simulink model "spoco12_100"  (R2013a)
settings: Solver=VariableStepDiscrete  SolverMode=SingleTasking  StartTime=0.0  StopTime=10.0  RelTol=1e-3
undefined symbols (not defined in the file or in its folder): casper_library_multipliers, cmult_4bit_em, pfb_coeff_gen_calc
libraries: xbsIndex_r4 x13471, casper_library_misc x184, xps_library x110, casper_library_delays x31
(part 3 of 135)

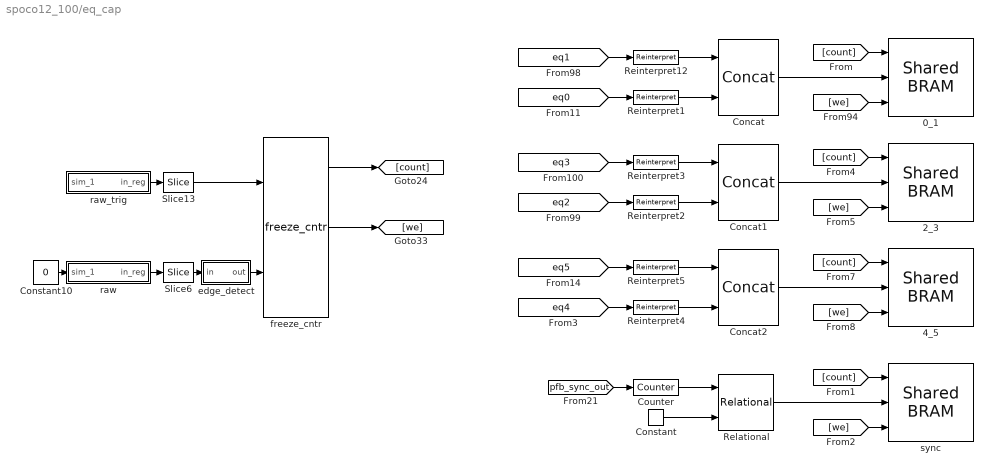
== system spoco12_100/eq_cap ==
  0_1 : xps_library/Shared BRAM  Tag=xps:bram  arith_type=Unsigned  addr_width=size+1  data_width=32  reg_prim_output=off  reg_core_output=off  optimization=Minimum_Area  data_bin_pt=0  init_vals=[1:2^10-1]  sample_rate=1
  2_3 : xps_library/Shared BRAM  Tag=xps:bram  arith_type=Unsigned  addr_width=size+1  data_width=32  reg_prim_output=off  reg_core_output=off  optimization=Minimum_Area  data_bin_pt=0  init_vals=[1:2^10-1]  sample_rate=1
  4_5 : xps_library/Shared BRAM  Tag=xps:bram  arith_type=Unsigned  addr_width=size+1  data_width=32  reg_prim_output=off  reg_core_output=off  optimization=Minimum_Area  data_bin_pt=0  init_vals=[1:2^10-1]  sample_rate=1
  Concat : xbsIndex_r4/Concat  num_inputs=2  dbl_ovrd=off  block_type=concat
  Concat1 : xbsIndex_r4/Concat  num_inputs=2  dbl_ovrd=off  block_type=concat
  Concat2 : xbsIndex_r4/Concat  num_inputs=2  dbl_ovrd=off  block_type=concat
  Constant : xbsIndex_r4/Constant  const=0  gui_display_data_type=Fixed-point  arith_type=Unsigned  n_bits=size  bin_pt=0  preci_type=Single  exp_width=8  frac_width=24  explicit_period=on  period=1  equ=P=C  opselect=C  inp2=PCIN>>17  opr=+  inp1=P  carry=CIN  dbl_ovrd=off  block_type=constant
  Constant10 : Constant  Value=0
  Counter : xbsIndex_r4/Counter  cnt_type=Free Running  cnt_to=Inf  operation=Up  start_count=0  cnt_by_val=1  arith_type=Unsigned  n_bits=size  bin_pt=0  load_pin=off  rst=on  en=off  explicit_period=on  period=1  use_behavioral_HDL=off  implementation=Fabric  dbl_ovrd=off  block_type=counter
  Reinterpret{1..5,12} (6 alike) : xbsIndex_r4/Reinterpret  force_arith_type=on  arith_type=Unsigned  force_bin_pt=on  bin_pt=0  block_type=reinterpret
  Relational : xbsIndex_r4/Relational  mode=a=b  op_type=Ufix  en=off  latency=0  dbl_ovrd=off  block_type=relational
  Slice13 : xbsIndex_r4/Slice  nbits=3  boolean_output=on  mode=Lower Bit Location + Width  bit1=0  base1=MSB of Input  bit0=0  base0=LSB of Input  dbl_ovrd=off  block_type=slice
  Slice6 : xbsIndex_r4/Slice  nbits=3  boolean_output=on  mode=Lower Bit Location + Width  bit1=0  base1=MSB of Input  bit0=0  base0=LSB of Input  dbl_ovrd=off  block_type=slice
  edge_detect : Subsystem  AncestorBlock=casper_library_misc/edge_detect  mask(edge_detect){edge=Both, polarity=Active High, x_in=[0 0.08 0.08 0.16 0.16 0.24 0.24 0.32 0.32 0.4], y_in=[-1 -1  1  1  1  1  1  1  1  1], x_out=[0.6 0.68 0.68 0.76 0.76 0.84 0.84 0.92 0.92 1], y_out=[-1 -1  1  1 -1 -1 -1 -1 -1 -1]}
      mask prompts: edge "Edge Type"; polarity "Output Polarity"; x_in "Input X Positions"; y_in "Input Y Positions"; x_out "Output X Positions"; y_out "Output Y Positions"
      mask help: Output is active for one-cycle after each edge of the specified type (i.e. rising, falling or both).
      mask init: same as spoco12_100/Sync/edge_detect1
      settings: AttributesFormatString=|
      | both edges
      | active high
      mask Help: Output is active for one-cycle after each edge of the specified type (i.e. rising, falling, or both).  Latency is zero.
      mask TypeOptions edge: Rising | Falling | Both
      mask TypeOptions polarity: Active High | Active Low
      mask Display:
      | plot(x_in_num,0.5+y_in_num*0.2);
      | plot(x_out_num,0.5+y_out_num*0.2);
  freeze_cntr : casper_library_misc/freeze_cntr  CounterBits=size+1
  raw : Subsystem  Tag=xps:sw_reg  AncestorBlock=xps_library/software register  mask(swreg){mode=one value, io_dir=From Processor, io_delay=0, sample_period=1, names=reg, bitwidths=32, arith_types=0, bin_pts=0, sim_port=on, show_format=off}
      mask prompts: io_dir "I/O direction"; io_delay "I/O delay"; sample_period "Sample period"; names "Name:"; bitwidths "Bitwidth:"; arith_types "Type (ufix=0, fix=1, bool=2):"; bin_pts "Binary pt:"; sim_port "Provide sim input/output?"; show_format "Print format string?"
      mask init:
      | swreg_init(gcb)
      settings: AttributesFormatString=1input
      mask TypeOptions mode: one value | fields of equal size | fields of arbitrary size
      mask Callback mode: swreg_cb(gcb);
      mask TypeOptions io_dir: To Processor | From Processor
      mask Callback io_dir:
      | mask_enables = get_param(gcb, 'MaskEnables');
      | mask_names = get_param(gcb, 'MaskNames');
      | if strcmp(get_param(gcb, 'io_dir'), 'To Processor'),
      |     mask_enables{ismember(mask_names, 'sample_period')} = 'off';
      | else
      |     mask_enables{ismember(mask_names, 'sample_period')} = 'on';
      | end
      | set_param(gcb, 'MaskEnables', mask_enables);
      mask Callback bitwidths:
      | swreg_maskcheck(gcb);
      | % blk = gcb;
      | % mode = get_param(blk, 'mode');
      | % current_widths = eval(get_param(blk, 'bitwidths'));
      | % if (strcmp(mode, 'one value') || strcmp(mode, 'fields of equal size')) && (length(current_widths) > 1),
      | %     error('Only one width may be specified for this mode.');
      | % elseif strcmp(mode, 'fields of arbitrary size')
      | %     current_names = textscan(strtrim(strrep(strrep(get_param(blk, 'names'), ']', ''), '[', '')), '%s');
      | %     current_names = current_names{1};
      | %     numios = length(current_names);
      | %     if length(current_widths) ~= numios,
      | %         error('%d field names specified, but %d widths?', numios, length(current_widths));
      | %     end
      | % end
      | % total_width = 0;
      | % for ctr = 1 : length(current_widths),
      | %     total_width = total_width + current_widths(ctr);
      | % end
      | % if total_width > 32,
      | %     error('Total width must be 32 or less, set to %d.', total_width);
      | % end
      mask Callback arith_types:
      | [numios, ~, ~, ~, current_types] = swreg_maskcheck(gcb);
      | % blk = gcb;
      | % mode = get_param(blk, 'mode');
      | % current_types = eval(get_param(blk, 'arith_types'));
      | % numios = length(current_types);
      | % if (strcmp(mode, 'one value') || strcmp(mode, 'fields of equal size')) && (length(current_types) > 1),
      | %     error('Only one type may be specified for this mode.');
      | % elseif strcmp(mode, 'fields of arbitrary size')
      | %     current_names = textscan(strtrim(strrep(strrep(get_param(blk, 'names'), ']', ''), '[', '')), '%s');
      | %     current_names = current_names{1};
      | %     numios = length(current_names);
      | %     if length(current_types) ~= numios,
      | %         error('%d field names specified, but %d types?', numios, length(current_types));
      | %     end
      | % end
      | problem = 0;
      | for ctr = 1 : numios,
      |     t = current_types(ctr);
      |     if (t < 0) || (t > 2),
      |         problem = t;
      |         ctr = numios + 1;
      |     end
      | end
      | if problem ~= 0,
      |     error('Type cannot be %i, must be 0, 1 or 2.', problem);
      | end
      mask Callback bin_pts:
      | swreg_maskcheck(gcb);
      | % blk = gcb;
      | % mode = get_param(blk, 'mode');
      | % current_bins = eval(get_param(blk, 'bin_pts'));
      | % if (strcmp(mode, 'one value') || strcmp(mode, 'fields of equal size')) && (length(current_bins) > 1),
      | %     error('Only one binary pt may be specified for this mode.');
      | % elseif strcmp(mode, 'fields of arbitrary size')
      | %     current_names = textscan(strtrim(strrep(strrep(get_param(blk, 'names'), ']', ''), '[', '')), '%s');
      | %     current_names = current_names{1};
      | %     numios = length(current_names);
      | %     if length(current_bins) ~= numios,
      | %         error('%d field names specified, but %d binary pts?', numios, length(current_bins));
      | %     end
      | % end
  raw_trig : Subsystem  Tag=xps:sw_reg  AncestorBlock=xps_library/software register  mask(swreg){mode=one value, io_dir=From Processor, io_delay=0, sample_period=1, names=reg, bitwidths=32, arith_types=0, bin_pts=0, sim_port=on, show_format=off}
      mask prompts: io_dir "I/O direction"; io_delay "I/O delay"; sample_period "Sample period"; names "Name:"; bitwidths "Bitwidth:"; arith_types "Type (ufix=0, fix=1, bool=2):"; bin_pts "Binary pt:"; sim_port "Provide sim input/output?"; show_format "Print format string?"
      mask init:
      | swreg_init(gcb)
      settings: AttributesFormatString=1input
      mask TypeOptions mode: one value | fields of equal size | fields of arbitrary size
      mask Callback mode: swreg_cb(gcb);
      mask TypeOptions io_dir: To Processor | From Processor
      mask Callback io_dir:
      | mask_enables = get_param(gcb, 'MaskEnables');
      | mask_names = get_param(gcb, 'MaskNames');
      | if strcmp(get_param(gcb, 'io_dir'), 'To Processor'),
      |     mask_enables{ismember(mask_names, 'sample_period')} = 'off';
      | else
      |     mask_enables{ismember(mask_names, 'sample_period')} = 'on';
      | end
      | set_param(gcb, 'MaskEnables', mask_enables);
      mask Callback bitwidths:
      | swreg_maskcheck(gcb);
      | % blk = gcb;
      | % mode = get_param(blk, 'mode');
      | % current_widths = eval(get_param(blk, 'bitwidths'));
      | % if (strcmp(mode, 'one value') || strcmp(mode, 'fields of equal size')) && (length(current_widths) > 1),
      | %     error('Only one width may be specified for this mode.');
      | % elseif strcmp(mode, 'fields of arbitrary size')
      | %     current_names = textscan(strtrim(strrep(strrep(get_param(blk, 'names'), ']', ''), '[', '')), '%s');
      | %     current_names = current_names{1};
      | %     numios = length(current_names);
      | %     if length(current_widths) ~= numios,
      | %         error('%d field names specified, but %d widths?', numios, length(current_widths));
      | %     end
      | % end
      | % total_width = 0;
      | % for ctr = 1 : length(current_widths),
      | %     total_width = total_width + current_widths(ctr);
      | % end
      | % if total_width > 32,
      | %     error('Total width must be 32 or less, set to %d.', total_width);
      | % end
      mask Callback arith_types:
      | [numios, ~, ~, ~, current_types] = swreg_maskcheck(gcb);
      | % blk = gcb;
      | % mode = get_param(blk, 'mode');
      | % current_types = eval(get_param(blk, 'arith_types'));
      | % numios = length(current_types);
      | % if (strcmp(mode, 'one value') || strcmp(mode, 'fields of equal size')) && (length(current_types) > 1),
      | %     error('Only one type may be specified for this mode.');
      | % elseif strcmp(mode, 'fields of arbitrary size')
      | %     current_names = textscan(strtrim(strrep(strrep(get_param(blk, 'names'), ']', ''), '[', '')), '%s');
      | %     current_names = current_names{1};
      | %     numios = length(current_names);
      | %     if length(current_types) ~= numios,
      | %         error('%d field names specified, but %d types?', numios, length(current_types));
      | %     end
      | % end
      | problem = 0;
      | for ctr = 1 : numios,
      |     t = current_types(ctr);
      |     if (t < 0) || (t > 2),
      |         problem = t;
      |         ctr = numios + 1;
      |     end
      | end
      | if problem ~= 0,
      |     error('Type cannot be %i, must be 0, 1 or 2.', problem);
      | end
      mask Callback bin_pts:
      | swreg_maskcheck(gcb);
      | % blk = gcb;
      | % mode = get_param(blk, 'mode');
      | % current_bins = eval(get_param(blk, 'bin_pts'));
      | % if (strcmp(mode, 'one value') || strcmp(mode, 'fields of equal size')) && (length(current_bins) > 1),
      | %     error('Only one binary pt may be specified for this mode.');
      | % elseif strcmp(mode, 'fields of arbitrary size')
      | %     current_names = textscan(strtrim(strrep(strrep(get_param(blk, 'names'), ']', ''), '[', '')), '%s');
      | %     current_names = current_names{1};
      | %     numios = length(current_names);
      | %     if length(current_bins) ~= numios,
      | %         error('%d field names specified, but %d binary pts?', numios, length(current_bins));
      | %     end
      | % end
  sync : xps_library/Shared BRAM  Tag=xps:bram  arith_type=Unsigned  addr_width=size+1  data_width=32  reg_prim_output=off  reg_core_output=off  optimization=Minimum_Area  data_bin_pt=0  init_vals=[1:2^10-1]  sample_rate=1
  wires:
  Constant/1 -> Relational/2
  Counter/1 -> Relational/1
  Relational/1 -> sync/2
  [pfb_sync_out] -> Counter/1
  [count] -> sync/1
  [we] -> sync/3
  raw/1(in_reg) -> Slice6/1
  freeze_cntr/1 -> [count]
  Slice6/1 -> edge_detect/1(in)
  freeze_cntr/2 -> [we]
  edge_detect/1(out) -> freeze_cntr/2
  raw_trig/1(in_reg) -> Slice13/1
  Slice13/1 -> freeze_cntr/1
  Constant10/1 -> raw/1(sim_1)
  Reinterpret1/1 -> Concat/2
  [eq1] -> Reinterpret12/1
  Reinterpret12/1 -> Concat/1
  Concat/1 -> 0_1/2
  [count] -> 0_1/1
  [we] -> 0_1/3
  [eq0] -> Reinterpret1/1
  Reinterpret2/1 -> Concat1/2
  Reinterpret3/1 -> Concat1/1
  Concat1/1 -> 2_3/2
  [count] -> 2_3/1
  [we] -> 2_3/3
  [eq2] -> Reinterpret2/1
  [eq3] -> Reinterpret3/1
  Reinterpret4/1 -> Concat2/2
  Reinterpret5/1 -> Concat2/1
  Concat2/1 -> 4_5/2
  [count] -> 4_5/1
  [we] -> 4_5/3
  [eq4] -> Reinterpret4/1
  [eq5] -> Reinterpret5/1

== system spoco12_100/eq_coeff ==
  sim_1 : Inport
  io_delay : xbsIndex_r4/Delay  rst=off  infoeditControl=Selection of Reset will increase slice count due to use of real FFs and instead of SRLs  en=off  latency=0  reg_retiming=on  dbl_ovrd=off  block_type=delay
  reint1 : xbsIndex_r4/Reinterpret  force_arith_type=on  arith_type=Unsigned  force_bin_pt=on  bin_pt=0  block_type=reinterpret
  slice_reg : xbsIndex_r4/Slice  nbits=32  boolean_output=off  mode=Lower Bit Location + Width  bit1=0  base1=MSB of Input  bit0=0  base0=LSB of Input  dbl_ovrd=off  block_type=slice
  spoco12_eq_coeff_user_data_out : xbsIndex_r4/Gateway In  gui_display_data_type=Fixed-point  arith_type=Unsigned  n_bits=32  bin_pt=0  preci_type=Single  exp_width=8  frac_width=24  rows=1  columns=1  quantization="Round  (unbiased: +/- Inf)"  overflow=Saturate  period=1  UseAsADC=off  ADCChannel='1'  interface=None  automatic_assignment=on  address_offset=hex2dec('00')  intf_description=''  timing_constraint=None  locs_specified=off  LOCs={}  io_standard={}  inherit_from_input=off  hdl_port=on  dbl_ovrd=off  block_type=gatewayin
  in_reg : Outport
  wires:
  spoco12_eq_coeff_user_data_out/1 -> io_delay/1
  sim_1/1 -> spoco12_eq_coeff_user_data_out/1
  io_delay/1 -> slice_reg/1
  slice_reg/1 -> reint1/1
  reint1/1 -> in_reg/1

== system spoco12_100/fft ==
  sync : Inport
  shift : Inport  Port=2
  pol0_in : Inport  Port=3
  pol1_in : Inport  Port=4
  pol2_in : Inport  Port=5
  pol3_in : Inport  Port=6
  pol4_in : Inport  Port=7
  pol5_in : Inport  Port=8
  pol6_in : Inport  Port=9
  pol7_in : Inport  Port=10
  pol8_in : Inport  Port=11
  pol9_in : Inport  Port=12
  pol10_in : Inport  Port=13
  pol11_in : Inport  Port=14
  fft_biplex_real_2x : Subsystem  Tag=casper:fft_biplex_real_2x  AncestorBlock=casper_library_ffts/fft_biplex_real_2x  mask(fft_biplex_real_2x){n_inputs=3, FFTSize=size, input_bit_width=18, bin_pt=17, coeff_bit_width=18, async=off, add_latency=add_z, mult_latency=mult_z, bram_latency=bram_z, conv_latency=cast_z, quantization=Round  (unbiased: +/- Inf), overflow=Saturate, delays_bit_limit=8, coeffs_bit_limit=8, coeff_sharing=on, coeff_decimation=on, max_fanout=4, mult_spec=2, bitgrowth=off, max_bits=19, hardcode_shifts=off, shift_schedule=[1                                      1], dsp48_adders=off}
      mask prompts: n_inputs "Number simultaneous inputs (4*?)"; FFTSize "Size of FFT: (2^? pts)"; input_bit_width "Input bit width"; bin_pt "Input binary point"; coeff_bit_width "Coefficient Bit Width"; async "Asynchronous operation"; add_latency "Add Latency"; mult_latency "Mult Latency"; bram_latency "BRAM Latency"; conv_latency "Convert latency"; quantization "Quantization Behavior"; overflow "Overflow Behavior"; delays_bit_limit "Number bits above which to implement stage's delays in BRAM (2^? bits)"; coeffs_bit_limit "Number bits above which to store stage's coefficients in BRAM (2^? bits)"; coeff_sharing "BRAM sharing in coeff storage"; coeff_decimation "Store a fraction of coeff factors where useful"; max_fanout "Maximum fanout"; mult_spec "Multiplier impl. (0=core, 1=embedded, 2=behavioural) (left=1st stage, or just one value)"; bitgrowth "Bit growth instead of shifting"; max_bits "Max bits to growth to"; hardcode_shifts "Hardcode shift schedule"; shift_schedule "Shift schedule"; dsp48_adders "DSP48 adders in butterfly"
      mask help: A real-sampled biplex FFT, with output demuxed by 2.
      mask init:
      | fft_biplex_real_2x_init(gcb, ...
      |     'n_inputs', n_inputs, ...
      |     'FFTSize', FFTSize, ...
      |     'input_bit_width', input_bit_width, ... 
      |     'bin_pt', bin_pt, ...
      |     'coeff_bit_width', coeff_bit_width, ...
      |     'async', async, ...
      |     'add_latency', add_latency, ...
      |     'mult_latency', mult_latency, ...
      |     'bram_latency', bram_latency, ...
      |     'conv_latency', conv_latency, ...
      |     'quantization', quantization, ...
      |     'overflow', overflow, ...
      |     'delays_bit_limit', delays_bit_limit, ...
      |     'coeffs_bit_limit', coeffs_bit_limit, ...
      |     'coeff_sharing', coeff_sharing, ...
      |     'coeff_decimation', coeff_decimation, ...
      |     'max_fanout', max_fanout, ...
      |     'mult_spec', mult_spec, ...
      |     'bitgrowth', bitgrowth, ...
      |     'max_bits', max_bits, ...
      |     'hardcode_shifts', hardcode_shifts, ...
      |     'shift_schedule', shift_schedule, ...
      |     'dsp48_adders', dsp48_adders);
      settings: AttributesFormatString=|
      | 10 stages
      | [18,18]
      | Round  (unbiased: +/- Inf)
      | Saturate
      mask Help: eval('xlWeb(''http://casper.berkeley.edu/wiki/Fft_biplex_real_2x'')')
      mask TypeOptions quantization: Truncate | Round  (unbiased: +/- Inf) | Round  (unbiased: Even Values)
      mask TypeOptions overflow: Wrap | Saturate | Error
      mask Callback hardcode_shifts:
      | hardcode_shifts = get_param(gcb, 'hardcode_shifts');
      | set_param_state(gcb, 'shift_schedule', hardcode_shifts);
      mask Callback dsp48_adders: fft_callback_dsp48_adders(gcb);
  sync_out : Outport
  pol02_out : Outport  Port=2
  pol13_out : Outport  Port=3
  pol46_out : Outport  Port=4
  pol57_out : Outport  Port=5
  pol810_out : Outport  Port=6
  pol911_out : Outport  Port=7
  of : Outport  Port=8
  wires:
  fft_biplex_real_2x/8(of) -> of/1
  shift/1 -> fft_biplex_real_2x/2(shift)
  sync/1 -> fft_biplex_real_2x/1(sync)
  fft_biplex_real_2x/1(sync_out) -> [sync_out], sync_out/1
  fft_biplex_real_2x/2(pol02_out) -> [pol02_out], pol02_out/1
  fft_biplex_real_2x/3(pol13_out) -> [pol13_out], pol13_out/1
  fft_biplex_real_2x/4(pol46_out) -> [pol46_out], pol46_out/1
  fft_biplex_real_2x/5(pol57_out) -> [pol57_out], pol57_out/1
  fft_biplex_real_2x/6(pol810_out) -> [pol810_out], pol810_out/1
  fft_biplex_real_2x/7(pol911_out) -> [pol911_out], pol911_out/1
  pol0_in/1 -> fft_biplex_real_2x/3(pol0_in)
  pol9_in/1 -> fft_biplex_real_2x/12(pol9_in)
  pol7_in/1 -> fft_biplex_real_2x/10(pol7_in)
  pol8_in/1 -> fft_biplex_real_2x/11(pol8_in)
  pol11_in/1 -> fft_biplex_real_2x/14(pol11_in)
  pol3_in/1 -> fft_biplex_real_2x/6(pol3_in)
  pol6_in/1 -> fft_biplex_real_2x/9(pol6_in)
  pol10_in/1 -> fft_biplex_real_2x/13(pol10_in)
  pol5_in/1 -> fft_biplex_real_2x/8(pol5_in)
  pol1_in/1 -> fft_biplex_real_2x/4(pol1_in)
  pol2_in/1 -> fft_biplex_real_2x/5(pol2_in)
  pol4_in/1 -> fft_biplex_real_2x/7(pol4_in)

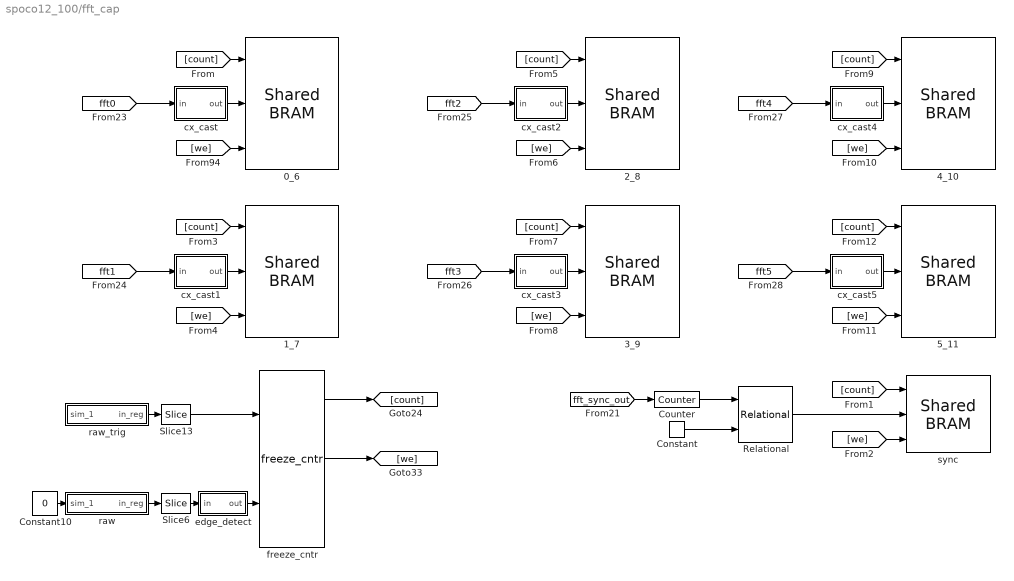
== system spoco12_100/fft_cap ==
  0_6 : xps_library/Shared BRAM  Tag=xps:bram  arith_type=Unsigned  addr_width=size+1  data_width=32  reg_prim_output=off  reg_core_output=off  optimization=Minimum_Area  data_bin_pt=0  init_vals=[1:2^10-1]  sample_rate=1
  1_7 : xps_library/Shared BRAM  Tag=xps:bram  arith_type=Unsigned  addr_width=size+1  data_width=32  reg_prim_output=off  reg_core_output=off  optimization=Minimum_Area  data_bin_pt=0  init_vals=[1:2^10-1]  sample_rate=1
  2_8 : xps_library/Shared BRAM  Tag=xps:bram  arith_type=Unsigned  addr_width=size+1  data_width=32  reg_prim_output=off  reg_core_output=off  optimization=Minimum_Area  data_bin_pt=0  init_vals=[1:2^10-1]  sample_rate=1
  3_9 : xps_library/Shared BRAM  Tag=xps:bram  arith_type=Unsigned  addr_width=size+1  data_width=32  reg_prim_output=off  reg_core_output=off  optimization=Minimum_Area  data_bin_pt=0  init_vals=[1:2^10-1]  sample_rate=1
  4_10 : xps_library/Shared BRAM  Tag=xps:bram  arith_type=Unsigned  addr_width=size+1  data_width=32  reg_prim_output=off  reg_core_output=off  optimization=Minimum_Area  data_bin_pt=0  init_vals=[1:2^10-1]  sample_rate=1
  5_11 : xps_library/Shared BRAM  Tag=xps:bram  arith_type=Unsigned  addr_width=size+1  data_width=32  reg_prim_output=off  reg_core_output=off  optimization=Minimum_Area  data_bin_pt=0  init_vals=[1:2^10-1]  sample_rate=1
  Constant : xbsIndex_r4/Constant  const=0  gui_display_data_type=Fixed-point  arith_type=Unsigned  n_bits=size  bin_pt=0  preci_type=Single  exp_width=8  frac_width=24  explicit_period=on  period=1  equ=P=C  opselect=C  inp2=PCIN>>17  opr=+  inp1=P  carry=CIN  dbl_ovrd=off  block_type=constant
  Constant10 : Constant  Value=0
  Counter : xbsIndex_r4/Counter  cnt_type=Free Running  cnt_to=Inf  operation=Up  start_count=0  cnt_by_val=1  arith_type=Unsigned  n_bits=size  bin_pt=0  load_pin=off  rst=on  en=off  explicit_period=on  period=1  use_behavioral_HDL=off  implementation=Fabric  dbl_ovrd=off  block_type=counter
  Relational : xbsIndex_r4/Relational  mode=a=b  op_type=Ufix  en=off  latency=0  dbl_ovrd=off  block_type=relational
  Slice13 : xbsIndex_r4/Slice  nbits=3  boolean_output=on  mode=Lower Bit Location + Width  bit1=0  base1=MSB of Input  bit0=0  base0=LSB of Input  dbl_ovrd=off  block_type=slice
  Slice6 : xbsIndex_r4/Slice  nbits=3  boolean_output=on  mode=Lower Bit Location + Width  bit1=0  base1=MSB of Input  bit0=0  base0=LSB of Input  dbl_ovrd=off  block_type=slice
  cx_cast : Subsystem  mask{in_bits=18, in_bp=17, out_bits=16, out_bp=15}
      mask prompts: in_bits "Input bits"; in_bp "Input binary point"; out_bits "Output bits"; out_bp "Output binary point"
  cx_cast1 : Subsystem  mask{in_bits=18, in_bp=17, out_bits=16, out_bp=15}
      mask prompts: in_bits "Input bits"; in_bp "Input binary point"; out_bits "Output bits"; out_bp "Output binary point"
  cx_cast2 : Subsystem  mask{in_bits=18, in_bp=17, out_bits=16, out_bp=15}
      mask prompts: in_bits "Input bits"; in_bp "Input binary point"; out_bits "Output bits"; out_bp "Output binary point"
  cx_cast3 : Subsystem  mask{in_bits=18, in_bp=17, out_bits=16, out_bp=15}
      mask prompts: in_bits "Input bits"; in_bp "Input binary point"; out_bits "Output bits"; out_bp "Output binary point"
  cx_cast4 : Subsystem  mask{in_bits=18, in_bp=17, out_bits=16, out_bp=15}
      mask prompts: in_bits "Input bits"; in_bp "Input binary point"; out_bits "Output bits"; out_bp "Output binary point"
  cx_cast5 : Subsystem  mask{in_bits=18, in_bp=17, out_bits=16, out_bp=15}
      mask prompts: in_bits "Input bits"; in_bp "Input binary point"; out_bits "Output bits"; out_bp "Output binary point"
  edge_detect : Subsystem  AncestorBlock=casper_library_misc/edge_detect  mask(edge_detect){edge=Both, polarity=Active High, x_in=[0 0.08 0.08 0.16 0.16 0.24 0.24 0.32 0.32 0.4], y_in=[-1 -1  1  1  1  1  1  1  1  1], x_out=[0.6 0.68 0.68 0.76 0.76 0.84 0.84 0.92 0.92 1], y_out=[-1 -1  1  1 -1 -1 -1 -1 -1 -1]}
      mask prompts: edge "Edge Type"; polarity "Output Polarity"; x_in "Input X Positions"; y_in "Input Y Positions"; x_out "Output X Positions"; y_out "Output Y Positions"
      mask help: Output is active for one-cycle after each edge of the specified type (i.e. rising, falling or both).
      mask init: same as spoco12_100/Sync/edge_detect1
      settings: AttributesFormatString=|
      | both edges
      | active high
      mask Help: Output is active for one-cycle after each edge of the specified type (i.e. rising, falling, or both).  Latency is zero.
      mask TypeOptions edge: Rising | Falling | Both
      mask TypeOptions polarity: Active High | Active Low
      mask Display:
      | plot(x_in_num,0.5+y_in_num*0.2);
      | plot(x_out_num,0.5+y_out_num*0.2);
  freeze_cntr : casper_library_misc/freeze_cntr  CounterBits=size+1
  raw : Subsystem  Tag=xps:sw_reg  AncestorBlock=xps_library/software register  mask(swreg){mode=one value, io_dir=From Processor, io_delay=0, sample_period=1, names=reg, bitwidths=32, arith_types=0, bin_pts=0, sim_port=on, show_format=off}
      mask prompts: io_dir "I/O direction"; io_delay "I/O delay"; sample_period "Sample period"; names "Name:"; bitwidths "Bitwidth:"; arith_types "Type (ufix=0, fix=1, bool=2):"; bin_pts "Binary pt:"; sim_port "Provide sim input/output?"; show_format "Print format string?"
      mask init:
      | swreg_init(gcb)
      settings: AttributesFormatString=1input
      mask TypeOptions mode: one value | fields of equal size | fields of arbitrary size
      mask Callback mode: swreg_cb(gcb);
      mask TypeOptions io_dir: To Processor | From Processor
      mask Callback io_dir:
      | mask_enables = get_param(gcb, 'MaskEnables');
      | mask_names = get_param(gcb, 'MaskNames');
      | if strcmp(get_param(gcb, 'io_dir'), 'To Processor'),
      |     mask_enables{ismember(mask_names, 'sample_period')} = 'off';
      | else
      |     mask_enables{ismember(mask_names, 'sample_period')} = 'on';
      | end
      | set_param(gcb, 'MaskEnables', mask_enables);
      mask Callback bitwidths:
      | swreg_maskcheck(gcb);
      | % blk = gcb;
      | % mode = get_param(blk, 'mode');
      | % current_widths = eval(get_param(blk, 'bitwidths'));
      | % if (strcmp(mode, 'one value') || strcmp(mode, 'fields of equal size')) && (length(current_widths) > 1),
      | %     error('Only one width may be specified for this mode.');
      | % elseif strcmp(mode, 'fields of arbitrary size')
      | %     current_names = textscan(strtrim(strrep(strrep(get_param(blk, 'names'), ']', ''), '[', '')), '%s');
      | %     current_names = current_names{1};
      | %     numios = length(current_names);
      | %     if length(current_widths) ~= numios,
      | %         error('%d field names specified, but %d widths?', numios, length(current_widths));
      | %     end
      | % end
      | % total_width = 0;
      | % for ctr = 1 : length(current_widths),
      | %     total_width = total_width + current_widths(ctr);
      | % end
      | % if total_width > 32,
      | %     error('Total width must be 32 or less, set to %d.', total_width);
      | % end
      mask Callback arith_types:
      | [numios, ~, ~, ~, current_types] = swreg_maskcheck(gcb);
      | % blk = gcb;
      | % mode = get_param(blk, 'mode');
      | % current_types = eval(get_param(blk, 'arith_types'));
      | % numios = length(current_types);
      | % if (strcmp(mode, 'one value') || strcmp(mode, 'fields of equal size')) && (length(current_types) > 1),
      | %     error('Only one type may be specified for this mode.');
      | % elseif strcmp(mode, 'fields of arbitrary size')
      | %     current_names = textscan(strtrim(strrep(strrep(get_param(blk, 'names'), ']', ''), '[', '')), '%s');
      | %     current_names = current_names{1};
      | %     numios = length(current_names);
      | %     if length(current_types) ~= numios,
      | %         error('%d field names specified, but %d types?', numios, length(current_types));
      | %     end
      | % end
      | problem = 0;
      | for ctr = 1 : numios,
      |     t = current_types(ctr);
      |     if (t < 0) || (t > 2),
      |         problem = t;
      |         ctr = numios + 1;
      |     end
      | end
      | if problem ~= 0,
      |     error('Type cannot be %i, must be 0, 1 or 2.', problem);
      | end
      mask Callback bin_pts:
      | swreg_maskcheck(gcb);
      | % blk = gcb;
      | % mode = get_param(blk, 'mode');
      | % current_bins = eval(get_param(blk, 'bin_pts'));
      | % if (strcmp(mode, 'one value') || strcmp(mode, 'fields of equal size')) && (length(current_bins) > 1),
      | %     error('Only one binary pt may be specified for this mode.');
      | % elseif strcmp(mode, 'fields of arbitrary size')
      | %     current_names = textscan(strtrim(strrep(strrep(get_param(blk, 'names'), ']', ''), '[', '')), '%s');
      | %     current_names = current_names{1};
      | %     numios = length(current_names);
      | %     if length(current_bins) ~= numios,
      | %         error('%d field names specified, but %d binary pts?', numios, length(current_bins));
      | %     end
      | % end
  raw_trig : Subsystem  Tag=xps:sw_reg  AncestorBlock=xps_library/software register  mask(swreg){mode=one value, io_dir=From Processor, io_delay=0, sample_period=1, names=reg, bitwidths=32, arith_types=0, bin_pts=0, sim_port=on, show_format=off}
      mask prompts: io_dir "I/O direction"; io_delay "I/O delay"; sample_period "Sample period"; names "Name:"; bitwidths "Bitwidth:"; arith_types "Type (ufix=0, fix=1, bool=2):"; bin_pts "Binary pt:"; sim_port "Provide sim input/output?"; show_format "Print format string?"
      mask init:
      | swreg_init(gcb)
      settings: AttributesFormatString=1input
      mask TypeOptions mode: one value | fields of equal size | fields of arbitrary size
      mask Callback mode: swreg_cb(gcb);
      mask TypeOptions io_dir: To Processor | From Processor
      mask Callback io_dir:
      | mask_enables = get_param(gcb, 'MaskEnables');
      | mask_names = get_param(gcb, 'MaskNames');
      | if strcmp(get_param(gcb, 'io_dir'), 'To Processor'),
      |     mask_enables{ismember(mask_names, 'sample_period')} = 'off';
      | else
      |     mask_enables{ismember(mask_names, 'sample_period')} = 'on';
      | end
      | set_param(gcb, 'MaskEnables', mask_enables);
      mask Callback bitwidths:
      | swreg_maskcheck(gcb);
      | % blk = gcb;
      | % mode = get_param(blk, 'mode');
      | % current_widths = eval(get_param(blk, 'bitwidths'));
      | % if (strcmp(mode, 'one value') || strcmp(mode, 'fields of equal size')) && (length(current_widths) > 1),
      | %     error('Only one width may be specified for this mode.');
      | % elseif strcmp(mode, 'fields of arbitrary size')
      | %     current_names = textscan(strtrim(strrep(strrep(get_param(blk, 'names'), ']', ''), '[', '')), '%s');
      | %     current_names = current_names{1};
      | %     numios = length(current_names);
      | %     if length(current_widths) ~= numios,
      | %         error('%d field names specified, but %d widths?', numios, length(current_widths));
      | %     end
      | % end
      | % total_width = 0;
      | % for ctr = 1 : length(current_widths),
      | %     total_width = total_width + current_widths(ctr);
      | % end
      | % if total_width > 32,
      | %     error('Total width must be 32 or less, set to %d.', total_width);
      | % end
      mask Callback arith_types:
      | [numios, ~, ~, ~, current_types] = swreg_maskcheck(gcb);
      | % blk = gcb;
      | % mode = get_param(blk, 'mode');
      | % current_types = eval(get_param(blk, 'arith_types'));
      | % numios = length(current_types);
      | % if (strcmp(mode, 'one value') || strcmp(mode, 'fields of equal size')) && (length(current_types) > 1),
      | %     error('Only one type may be specified for this mode.');
      | % elseif strcmp(mode, 'fields of arbitrary size')
      | %     current_names = textscan(strtrim(strrep(strrep(get_param(blk, 'names'), ']', ''), '[', '')), '%s');
      | %     current_names = current_names{1};
      | %     numios = length(current_names);
      | %     if length(current_types) ~= numios,
      | %         error('%d field names specified, but %d types?', numios, length(current_types));
      | %     end
      | % end
      | problem = 0;
      | for ctr = 1 : numios,
      |     t = current_types(ctr);
      |     if (t < 0) || (t > 2),
      |         problem = t;
      |         ctr = numios + 1;
      |     end
      | end
      | if problem ~= 0,
      |     error('Type cannot be %i, must be 0, 1 or 2.', problem);
      | end
      mask Callback bin_pts:
      | swreg_maskcheck(gcb);
      | % blk = gcb;
      | % mode = get_param(blk, 'mode');
      | % current_bins = eval(get_param(blk, 'bin_pts'));
      | % if (strcmp(mode, 'one value') || strcmp(mode, 'fields of equal size')) && (length(current_bins) > 1),
      | %     error('Only one binary pt may be specified for this mode.');
      | % elseif strcmp(mode, 'fields of arbitrary size')
      | %     current_names = textscan(strtrim(strrep(strrep(get_param(blk, 'names'), ']', ''), '[', '')), '%s');
      | %     current_names = current_names{1};
      | %     numios = length(current_names);
      | %     if length(current_bins) ~= numios,
      | %         error('%d field names specified, but %d binary pts?', numios, length(current_bins));
      | %     end
      | % end
  sync : xps_library/Shared BRAM  Tag=xps:bram  arith_type=Unsigned  addr_width=size+1  data_width=32  reg_prim_output=off  reg_core_output=off  optimization=Minimum_Area  data_bin_pt=0  init_vals=[1:2^10-1]  sample_rate=1
  wires:
  Constant/1 -> Relational/2
  Counter/1 -> Relational/1
  Relational/1 -> sync/2
  [fft_sync_out] -> Counter/1
  [count] -> sync/1
  [we] -> sync/3
  raw/1(in_reg) -> Slice6/1
  freeze_cntr/1 -> [count]
  Slice6/1 -> edge_detect/1(in)
  freeze_cntr/2 -> [we]
  edge_detect/1(out) -> freeze_cntr/2
  raw_trig/1(in_reg) -> Slice13/1
  Slice13/1 -> freeze_cntr/1
  Constant10/1 -> raw/1(sim_1)
  [count] -> 0_6/1
  [we] -> 0_6/3
  [fft0] -> cx_cast/1(in)
  cx_cast/1(out) -> 0_6/2
  [count] -> 1_7/1
  [we] -> 1_7/3
  [fft1] -> cx_cast1/1(in)
  cx_cast1/1(out) -> 1_7/2
  [count] -> 2_8/1
  [we] -> 2_8/3
  [fft2] -> cx_cast2/1(in)
  cx_cast2/1(out) -> 2_8/2
  [count] -> 3_9/1
  [we] -> 3_9/3
  [fft3] -> cx_cast3/1(in)
  cx_cast3/1(out) -> 3_9/2
  [count] -> 4_10/1
  [we] -> 4_10/3
  [fft4] -> cx_cast4/1(in)
  cx_cast4/1(out) -> 4_10/2
  [count] -> 5_11/1
  [we] -> 5_11/3
  [fft5] -> cx_cast5/1(in)
  cx_cast5/1(out) -> 5_11/2

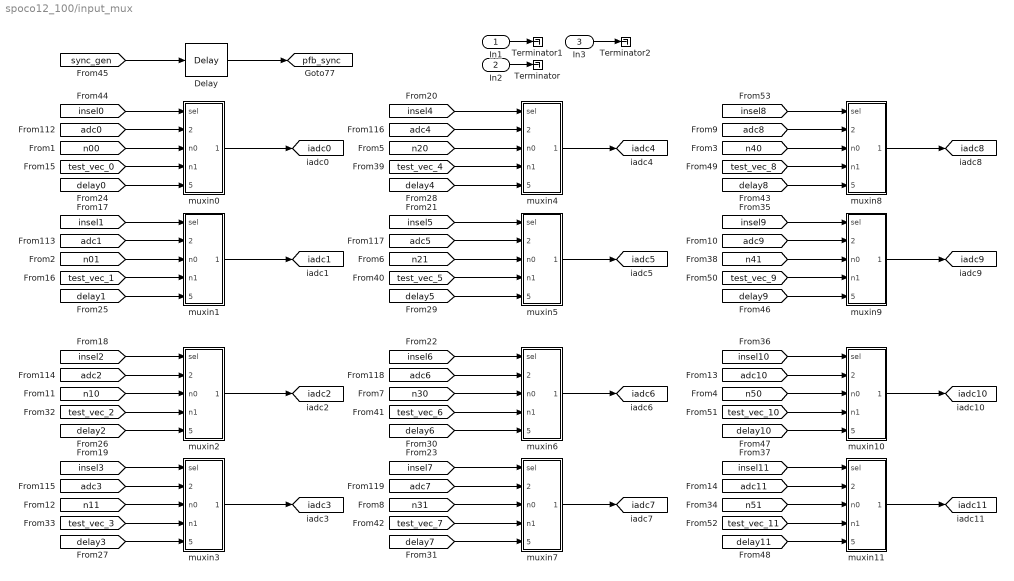
== system spoco12_100/input_mux ==
  In1 : Inport
  In2 : Inport  Port=2
  In3 : Inport  Port=3
  Delay : xbsIndex_r4/Delay  rst=off  infoeditControl=Selection of Reset will increase slice count due to use of real FFs and instead of SRLs  en=off  latency=2  reg_retiming=off  dbl_ovrd=off  block_type=delay
  Terminator : Terminator
  Terminator1 : Terminator
  Terminator2 : Terminator
  muxin0 : Subsystem
  muxin1 : Subsystem
  muxin10 : Subsystem
  muxin11 : Subsystem
  muxin2 : Subsystem
  muxin3 : Subsystem
  muxin4 : Subsystem
  muxin5 : Subsystem
  muxin6 : Subsystem
  muxin7 : Subsystem
  muxin8 : Subsystem
  muxin9 : Subsystem
  tag scope: iadc0=global, iadc10=global, iadc11=global, iadc1=global, iadc2=global, iadc3=global, iadc4=global, iadc5=global, iadc6=global, iadc7=global, iadc8=global, iadc9=global, pfb_sync=global
  wires:
  [insel0] -> muxin0/1(sel)
  [adc0] -> muxin0/2(adc)
  [n00] -> muxin0/3(n0)
  [delay0] -> muxin0/5(delay)
  [insel1] -> muxin1/1(sel)
  [adc1] -> muxin1/2(adc)
  [delay1] -> muxin1/5(delay)
  [insel2] -> muxin2/1(sel)
  [adc2] -> muxin2/2(adc)
  [n10] -> muxin2/3(n0)
  [delay2] -> muxin2/5(delay)
  [insel3] -> muxin3/1(sel)
  [adc3] -> muxin3/2(adc)
  [delay3] -> muxin3/5(delay)
  [insel4] -> muxin4/1(sel)
  [adc4] -> muxin4/2(adc)
  [n20] -> muxin4/3(n0)
  [delay4] -> muxin4/5(delay)
  [insel5] -> muxin5/1(sel)
  [adc5] -> muxin5/2(adc)
  [delay5] -> muxin5/5(delay)
  [insel6] -> muxin6/1(sel)
  [adc6] -> muxin6/2(adc)
  [n30] -> muxin6/3(n0)
  [delay6] -> muxin6/5(delay)
  [insel7] -> muxin7/1(sel)
  [adc7] -> muxin7/2(adc)
  [delay7] -> muxin7/5(delay)
  [sync_gen] -> Delay/1
  Delay/1 -> [pfb_sync]
  In1/1 -> Terminator1/1
  In2/1 -> Terminator/1
  [insel8] -> muxin8/1(sel)
  [adc8] -> muxin8/2(adc)
  [n40] -> muxin8/3(n0)
  [delay8] -> muxin8/5(delay)
  [insel9] -> muxin9/1(sel)
  [adc9] -> muxin9/2(adc)
  [delay9] -> muxin9/5(delay)
  [insel10] -> muxin10/1(sel)
  [adc10] -> muxin10/2(adc)
  [n50] -> muxin10/3(n0)
  [delay10] -> muxin10/5(delay)
  [insel11] -> muxin11/1(sel)
  [adc11] -> muxin11/2(adc)
  [delay11] -> muxin11/5(delay)
  muxin0/1(out) -> [iadc0]
  muxin1/1(out) -> [iadc1]
  muxin2/1(out) -> [iadc2]
  muxin3/1(out) -> [iadc3]
  muxin4/1(out) -> [iadc4]
  muxin5/1(out) -> [iadc5]
  muxin6/1(out) -> [iadc6]
  muxin7/1(out) -> [iadc7]
  muxin8/1(out) -> [iadc8]
  muxin9/1(out) -> [iadc9]
  muxin10/1(out) -> [iadc10]
  muxin11/1(out) -> [iadc11]
  [n01] -> muxin1/3(n0)
  [n11] -> muxin3/3(n0)
  [n21] -> muxin5/3(n0)
  [n31] -> muxin7/3(n0)
  [n41] -> muxin9/3(n0)
  [n51] -> muxin11/3(n0)
  In3/1 -> Terminator2/1
  [test_vec_0] -> muxin0/4(n1)
  [test_vec_1] -> muxin1/4(n1)
  [test_vec_2] -> muxin2/4(n1)
  [test_vec_3] -> muxin3/4(n1)
  [test_vec_4] -> muxin4/4(n1)
  [test_vec_5] -> muxin5/4(n1)
  [test_vec_6] -> muxin6/4(n1)
  [test_vec_7] -> muxin7/4(n1)
  [test_vec_8] -> muxin8/4(n1)
  [test_vec_9] -> muxin9/4(n1)
  [test_vec_10] -> muxin10/4(n1)
  [test_vec_11] -> muxin11/4(n1)

== system spoco12_100/insel ==
  note: insel is a 32 bit input. every 4 bits represents a
      | selection input in the mux subsystem block. The inputs
      | are as follows:0=adc, 1=noise0, 2=noise1, 3=constant (0)
  BitBasher1 : xbsIndex_r4/BitBasher  bitexpr=|  display_expr=off  sr_1=insel8  arith_type1=Unsigned  bin_pt1=0  sr_2=insel9  arith_type2=Unsigned  bin_pt2=0  sr_3=insel10  arith_type3=Unsigned  bin_pt3=0  sr_4=insel11  arith_type4=Unsigned  bin_pt4=0  dbl_ovrd=off  block_type=bitbasher
      | insel8={insel[17:16]}
      | insel9={insel[19:18]}
      | insel10={insel[21:20]}
      | insel11={insel[23:22]}
  BitBasher4 : xbsIndex_r4/BitBasher  bitexpr=|  display_expr=off  sr_1=insel0  arith_type1=Unsigned  bin_pt1=0  sr_2=insel1  arith_type2=Unsigned  bin_pt2=0  sr_3=insel2  arith_type3=Unsigned  bin_pt3=0  sr_4=insel3  arith_type4=Unsigned  bin_pt4=0  dbl_ovrd=off  block_type=bitbasher
      | insel0={insel[1:0]}
      | insel1={insel[3:2]}
      | insel2={insel[5:4]}
      | insel3={insel[7:6]}
  BitBasher5 : xbsIndex_r4/BitBasher  bitexpr=|  display_expr=off  sr_1=insel4  arith_type1=Unsigned  bin_pt1=0  sr_2=insel5  arith_type2=Unsigned  bin_pt2=0  sr_3=insel6  arith_type3=Unsigned  bin_pt3=0  sr_4=insel7  arith_type4=Unsigned  bin_pt4=0  dbl_ovrd=off  block_type=bitbasher
      | insel4={insel[9:8]}
      | insel5={insel[11:10]}
      | insel6={insel[13:12]}
      | insel7={insel[15:14]}
  Constant : Constant  Value=858862385
  insel_data : Subsystem  Tag=xps:sw_reg  AncestorBlock=xps_library/software register  mask(swreg){mode=one value, io_dir=From Processor, io_delay=0, sample_period=1, names=reg, bitwidths=32, arith_types=0, bin_pts=0, sim_port=on, show_format=off}
      mask prompts: io_dir "I/O direction"; io_delay "I/O delay"; sample_period "Sample period"; names "Name:"; bitwidths "Bitwidth:"; arith_types "Type (ufix=0, fix=1, bool=2):"; bin_pts "Binary pt:"; sim_port "Provide sim input/output?"; show_format "Print format string?"
      mask init:
      | swreg_init(gcb)
      settings: AttributesFormatString=1input
      mask TypeOptions mode: one value | fields of equal size | fields of arbitrary size
      mask Callback mode: swreg_cb(gcb);
      mask TypeOptions io_dir: To Processor | From Processor
      mask Callback io_dir:
      | mask_enables = get_param(gcb, 'MaskEnables');
      | mask_names = get_param(gcb, 'MaskNames');
      | if strcmp(get_param(gcb, 'io_dir'), 'To Processor'),
      |     mask_enables{ismember(mask_names, 'sample_period')} = 'off';
      | else
      |     mask_enables{ismember(mask_names, 'sample_period')} = 'on';
      | end
      | set_param(gcb, 'MaskEnables', mask_enables);
      mask Callback bitwidths:
      | swreg_maskcheck(gcb);
      | % blk = gcb;
      | % mode = get_param(blk, 'mode');
      | % current_widths = eval(get_param(blk, 'bitwidths'));
      | % if (strcmp(mode, 'one value') || strcmp(mode, 'fields of equal size')) && (length(current_widths) > 1),
      | %     error('Only one width may be specified for this mode.');
      | % elseif strcmp(mode, 'fields of arbitrary size')
      | %     current_names = textscan(strtrim(strrep(strrep(get_param(blk, 'names'), ']', ''), '[', '')), '%s');
      | %     current_names = current_names{1};
      | %     numios = length(current_names);
      | %     if length(current_widths) ~= numios,
      | %         error('%d field names specified, but %d widths?', numios, length(current_widths));
      | %     end
      | % end
      | % total_width = 0;
      | % for ctr = 1 : length(current_widths),
      | %     total_width = total_width + current_widths(ctr);
      | % end
      | % if total_width > 32,
      | %     error('Total width must be 32 or less, set to %d.', total_width);
      | % end
      mask Callback arith_types:
      | [numios, ~, ~, ~, current_types] = swreg_maskcheck(gcb);
      | % blk = gcb;
      | % mode = get_param(blk, 'mode');
      | % current_types = eval(get_param(blk, 'arith_types'));
      | % numios = length(current_types);
      | % if (strcmp(mode, 'one value') || strcmp(mode, 'fields of equal size')) && (length(current_types) > 1),
      | %     error('Only one type may be specified for this mode.');
      | % elseif strcmp(mode, 'fields of arbitrary size')
      | %     current_names = textscan(strtrim(strrep(strrep(get_param(blk, 'names'), ']', ''), '[', '')), '%s');
      | %     current_names = current_names{1};
      | %     numios = length(current_names);
      | %     if length(current_types) ~= numios,
      | %         error('%d field names specified, but %d types?', numios, length(current_types));
      | %     end
      | % end
      | problem = 0;
      | for ctr = 1 : numios,
      |     t = current_types(ctr);
      |     if (t < 0) || (t > 2),
      |         problem = t;
      |         ctr = numios + 1;
      |     end
      | end
      | if problem ~= 0,
      |     error('Type cannot be %i, must be 0, 1 or 2.', problem);
      | end
      mask Callback bin_pts:
      | swreg_maskcheck(gcb);
      | % blk = gcb;
      | % mode = get_param(blk, 'mode');
      | % current_bins = eval(get_param(blk, 'bin_pts'));
      | % if (strcmp(mode, 'one value') || strcmp(mode, 'fields of equal size')) && (length(current_bins) > 1),
      | %     error('Only one binary pt may be specified for this mode.');
      | % elseif strcmp(mode, 'fields of arbitrary size')
      | %     current_names = textscan(strtrim(strrep(strrep(get_param(blk, 'names'), ']', ''), '[', '')), '%s');
      | %     current_names = current_names{1};
      | %     numios = length(current_names);
      | %     if length(current_bins) ~= numios,
      | %         error('%d field names specified, but %d binary pts?', numios, length(current_bins));
      | %     end
      | % end
  tag scope: insel0=global, insel10=global, insel11=global, insel1=global, insel2=global, insel3=global, insel4=global, insel5=global, insel6=global, insel7=global, insel8=global, insel9=global
  wires:
  Constant/1 -> insel_data/1(sim_1)
  BitBasher4/1 -> [insel0]
  BitBasher4/2 -> [insel1]
  BitBasher4/3 -> [insel2]
  BitBasher4/4 -> [insel3]
  BitBasher5/1 -> [insel4]
  BitBasher5/2 -> [insel5]
  BitBasher5/3 -> [insel6]
  BitBasher5/4 -> [insel7]
  BitBasher1/1 -> [insel8]
  BitBasher1/2 -> [insel9]
  BitBasher1/3 -> [insel10]
  BitBasher1/4 -> [insel11]
  insel_data/1(in_reg) -> BitBasher4/1, BitBasher1/1, BitBasher5/1
